simulink model "non_linear_pid_250120"  (R2018b)
settings: Solver=VariableStepAuto  StartTime=0.0  StopTime=10.0  RelTol=1e-3
settings Model: Creator=Paweł Tymiński  LastModifiedBy=Paweł Tymiński

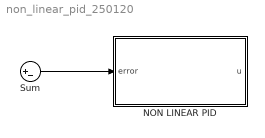
== system non_linear_pid_250120 ==
  NON LINEAR PID : Subsystem
  Sum : Sum  Inputs=|+-
  wires:
  Sum/1 -> NON LINEAR PID/1(error)

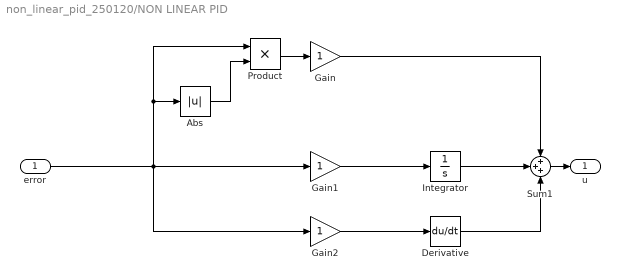
== system non_linear_pid_250120/NON LINEAR PID ==
  error : Inport
  Abs : Abs
  Derivative : Derivative
  Gain : Gain
  Gain1 : Gain
  Gain2 : Gain
  Integrator : Integrator
  Product : Product
  Sum1 : Sum  Inputs=+++
  u : Outport
  wires:
  Product/1 -> Gain/1
  Derivative/1 -> Sum1/3
  Integrator/1 -> Sum1/2
  error/1 -> Gain2/1, Gain1/1, Abs/1, Product/1
  Gain2/1 -> Derivative/1
  Abs/1 -> Product/2
  Gain/1 -> Sum1/1
  Gain1/1 -> Integrator/1
  Sum1/1 -> u/1
